simulink library "evironmentEstimation_lib"  (R2018b)
settings: Solver=VariableStepAuto  StartTime=0.0  StopTime=10.0  RelTol=1e-3
undefined symbols (not defined in the file or in its folder): fswParams
libraries: groundpass_predict_lib x1, magField_lib x1, sgp4_lib_fsw x1, sunVectorEclipse_lib x1, time_coord_rotations_lib x1
settings Model: Creator=devantormey  LastModifiedBy=aact_

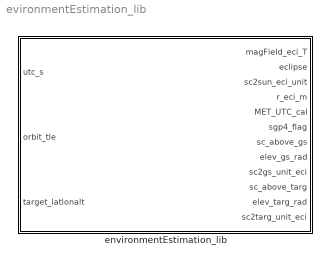
== system evironmentEstimation_lib ==
  environmentEstimation_lib : Subsystem  TreatAsAtomicUnit=on

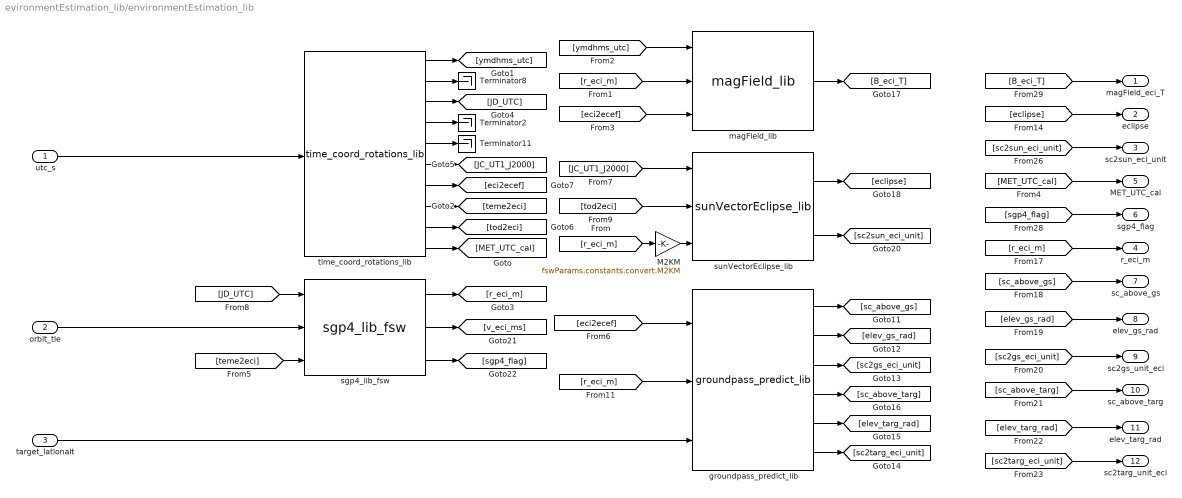
== system evironmentEstimation_lib/environmentEstimation_lib ==
  utc_s : Inport
  orbit_tle : Inport  Port=2
  target_latlonalt : Inport  Port=3
  M2KM : Gain  Gain=fswParams.constants.convert.M2KM
  Terminator11 : Terminator
  Terminator2 : Terminator
  Terminator8 : Terminator
  groundpass_predict_lib : groundpass_predict_lib/groundpass_predict_lib  SystemSampleTime=-1
  magField_lib : magField_lib/magField_lib  SystemSampleTime=-1
      link override Rate Transition2: InitialCondition=0
  sgp4_lib_fsw : sgp4_lib_fsw/sgp4_lib_fsw  SystemSampleTime=-1
  sunVectorEclipse_lib : sunVectorEclipse_lib/sunVectorEclipse_lib  SystemSampleTime=-1
  time_coord_rotations_lib : time_coord_rotations_lib/time_coord_rotations_lib  time_offset=fswParams.sensors.time_offset
  magField_eci_T : Outport
  eclipse : Outport  Port=2
  sc2sun_eci_unit : Outport  Port=3
  r_eci_m : Outport  Port=4
  MET_UTC_cal : Outport  Port=5
  sgp4_flag : Outport  Port=6
  sc_above_gs : Outport  Port=7
  elev_gs_rad : Outport  Port=8
  sc2gs_unit_eci : Outport  Port=9
  sc_above_targ : Outport  Port=10
  elev_targ_rad : Outport  Port=11
  sc2targ_unit_eci : Outport  Port=12
  wires:
  sgp4_lib_fsw/1 -> [r_eci_m]
  [r_eci_m] -> magField_lib/2
  [r_eci_m] -> M2KM/1
  [JC_UT1_J2000] -> sunVectorEclipse_lib/1
  orbit_tle/1 -> sgp4_lib_fsw/2
  [ymdhms_utc] -> magField_lib/1
  [eci2ecef] -> magField_lib/3
  time_coord_rotations_lib/7 -> [eci2ecef]
  time_coord_rotations_lib/8 -> [teme2eci]
  [teme2eci] -> sgp4_lib_fsw/3
  [r_eci_m] -> groundpass_predict_lib/2
  [JD_UTC] -> sgp4_lib_fsw/1
  target_latlonalt/1 -> groundpass_predict_lib/3
  [r_eci_m] -> r_eci_m/1
  groundpass_predict_lib/1 -> [sc_above_gs]
  groundpass_predict_lib/2 -> [elev_gs_rad]
  groundpass_predict_lib/3 -> [sc2gs_eci_unit]
  groundpass_predict_lib/4 -> [sc_above_targ]
  groundpass_predict_lib/5 -> [elev_targ_rad]
  groundpass_predict_lib/6 -> [sc2targ_eci_unit]
  sunVectorEclipse_lib/1 -> [eclipse]
  sunVectorEclipse_lib/2 -> [sc2sun_eci_unit]
  [sc_above_gs] -> sc_above_gs/1
  [elev_gs_rad] -> elev_gs_rad/1
  [sc2gs_eci_unit] -> sc2gs_unit_eci/1
  [sc_above_targ] -> sc_above_targ/1
  [elev_targ_rad] -> elev_targ_rad/1
  [sc2targ_eci_unit] -> sc2targ_unit_eci/1
  [sc2sun_eci_unit] -> sc2sun_eci_unit/1
  [eclipse] -> eclipse/1
  magField_lib/1 -> [B_eci_T]
  sgp4_lib_fsw/2 -> [v_eci_ms]
  [MET_UTC_cal] -> MET_UTC_cal/1
  sgp4_lib_fsw/3 -> [sgp4_flag]
  [sgp4_flag] -> sgp4_flag/1
  [B_eci_T] -> magField_eci_T/1
  time_coord_rotations_lib/1 -> [ymdhms_utc]
  time_coord_rotations_lib/2 -> Terminator8/1
  time_coord_rotations_lib/6 -> [JC_UT1_J2000]
  time_coord_rotations_lib/5 -> Terminator11/1
  time_coord_rotations_lib/3 -> [JD_UTC]
  time_coord_rotations_lib/4 -> Terminator2/1
  time_coord_rotations_lib/9 -> [tod2eci]
  [tod2eci] -> sunVectorEclipse_lib/2
  M2KM/1 -> sunVectorEclipse_lib/3
  [eci2ecef] -> groundpass_predict_lib/1
  utc_s/1 -> time_coord_rotations_lib/1
  time_coord_rotations_lib/10 -> [MET_UTC_cal]
